simulink model "LAB_07_SIM_GG_SRP"  (R2022b)
settings: Solver=ode8  StartTime=0.0  StopTime=10000  FixedStep=0.05  RelTol=1e-3
values from neighbouring files (symbols this model uses):
  a = 16371e+3    (= 16371000)    [lab_07_MAT.m]
  A0 = diag([1 1 1])    [LAB_04_17_OCT_MAT_KIN.m]    (also in LAB_05_24_OCT_MAT_KIN_COSDIR.m; LAB_06.m = A_target_fun(0); core_attitude_test.m = eye(3,3); lab_07_MAT.m)
  A_B1 = 2e-2    (= 0.02)    [lab_07_MAT.m]
  A_B2 = 6e-2    (= 0.06)    [lab_07_MAT.m]
  A_B3 = 2e-2    (= 0.02)    [lab_07_MAT.m]
  A_B4 = 6e-2    (= 0.06)    [lab_07_MAT.m]
  A_B5 = 3e-2    (= 0.03)    [lab_07_MAT.m]
  A_B6 = 3e-2    (= 0.03)    [lab_07_MAT.m]
  A_P1 = 12e-2    (= 0.12)    [lab_07_MAT.m]
  A_P2 = 12e-2    (= 0.12)    [lab_07_MAT.m]
  A_P3 = 12e-2    (= 0.12)    [lab_07_MAT.m]
  A_P4 = 12e-2    (= 0.12)    [lab_07_MAT.m]
  ang = deg2rad(11.5)    [lab_07_MAT.m]
  e = 0    [lab_07_MAT.m]
  G = 6.67430e-11    (= 6.6743e-11)    [LAB_06.m]    (also in lab_07_MAT.m)
  g_1_0 = -29404.8    [lab_07_MAT.m]
  g_1_1 = -1450.9    [lab_07_MAT.m]
  h_1_1 = 4652.5    [lab_07_MAT.m]
  i = char('pippo')    [LAB_01_19_SEPT.m]    (also in lab_07_MAT.m = 0.1)
  I = [Ix 0 0 ... (first row only)    [LAB_03_3_OCT_MAT_EUL_2_VERIFICATION.m]    (also in LAB_03_3_OCT_MAT_EUL_DOUBLESPIN.m = diag([Ix, Iy, Iz]); LAB_03_3_OCT_MAT_EUL_SPINAXIS.m = diag([Ix, Iy, Iz]); LAB_03_3_OCT_MAT_EUL_VECT.m; LAB_04_17_OCT_MAT_KIN.m)
  j_B = [0.01; 0.05; 0.01]    [lab_07_MAT.m]
  Mt = 5.972e+24    [LAB_06.m]    (also in lab_07_MAT.m)
  N_B1 = [1,0,0]'    [lab_07_MAT.m]
  N_B2 = [0,1,0]'    [lab_07_MAT.m]
  N_B3 = [-1,0,0]'    [lab_07_MAT.m]
  N_B4 = [0,-1,0]'    [lab_07_MAT.m]
  N_B5 = [0,0,1]'    [lab_07_MAT.m]
  N_B6 = [0,0,-1]    [lab_07_MAT.m]
  N_P1 = [0,0,1]    [lab_07_MAT.m]
  N_P2 = [0,0,-1]    [lab_07_MAT.m]
  N_P3 = [0,0,1]    [lab_07_MAT.m]
  N_P4 = [0,0,-1]    [lab_07_MAT.m]
  n_rot = 0.0012    [lab_07_MAT.m]
  n_sun = 2*pi/T    (= 1.99238499086e-07)    [lab_07_MAT.m]
  om_0 = [om_x0, om_y0, om_z0]    [LAB_03_3_OCT_MAT_EUL.m]    (also in LAB_03_3_OCT_MAT_EUL_2_VERIFICATION.m = [om_x0; om_y0; om_z0]; LAB_03_3_OCT_MAT_EUL_DOUBLESPIN.m = [om_x0; om_y0; om_z0]; LAB_03_3_OCT_MAT_EUL_SPINAXIS.m = [om_x0; om_y0; om_z0]; LAB_03_3_OCT_MAT_EUL_VECT.m = [om_x0; om_y0; om_z0])
  om_target = [0; 0; n]    [LAB_06.m]    (also in lab_07_MAT.m)
  P = [Px, Py, Pz]    [LAB_03_3_OCT_MAT_EUL_VECT.m]    (also in lab_07_MAT.m = 4.52666666667e-06)
  R = 6.371e+6 + H    (= 6381000)    [LAB_06.m]    (also in lab_07_MAT.m = 6378000)
  r_B1 = 1e-2*[15,0,0]    [lab_07_MAT.m]
  r_B2 = 1e-2*[0,5,0]    [lab_07_MAT.m]
  r_B3 = 1e-2*[-15,0,0]    [lab_07_MAT.m]
  r_B4 = 1e-2*[0,-5,0]    [lab_07_MAT.m]
  r_B5 = 1e-2*[0,0,10]    [lab_07_MAT.m]
  r_B6 = 1e-2*[0,0,-10]    [lab_07_MAT.m]
  r_P1 = 1e-2*[0,20,10]    [lab_07_MAT.m]
  r_P2 = 1e-2*[0,20,10]    [lab_07_MAT.m]
  r_P3 = 1e-2*[0,-20,10]    [lab_07_MAT.m]
  r_P4 = 1e-2*[0,-20,10]    [lab_07_MAT.m]
  r_sun = 149597870000    [lab_07_MAT.m]
  rho_d = 0.1    [lab_07_MAT.m]
  rho_sB = 0.5    [lab_07_MAT.m]
  rho_sP = 0.5    [lab_07_MAT.m]
  rot_E = 7.29e-5    (= 7.29e-05)    [lab_07_MAT.m]
  theta_0 = 3/2 * pi    (= 4.71238898038)    [lab_07_MAT.m]
libraries: matrix_library x17, sharedutil x3, vrlib x1
(part 1 of 2)
settings Model: Creator=maria  LastModifiedBy=maria
settings OptimizationCC: BlockReduction=off  DefaultParameterBehavior=Inlined  BufferReuse=off

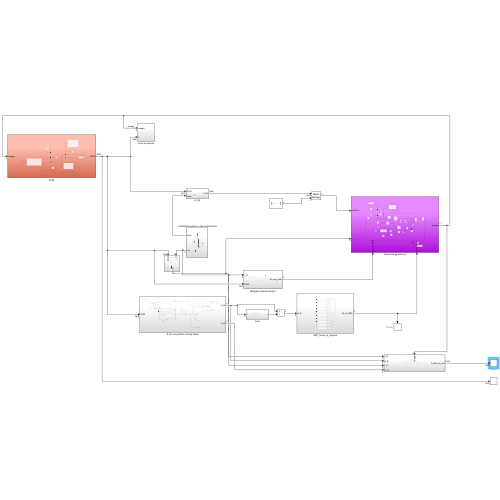
[thumbnail: Simulink's stored preview of the top-level diagram]
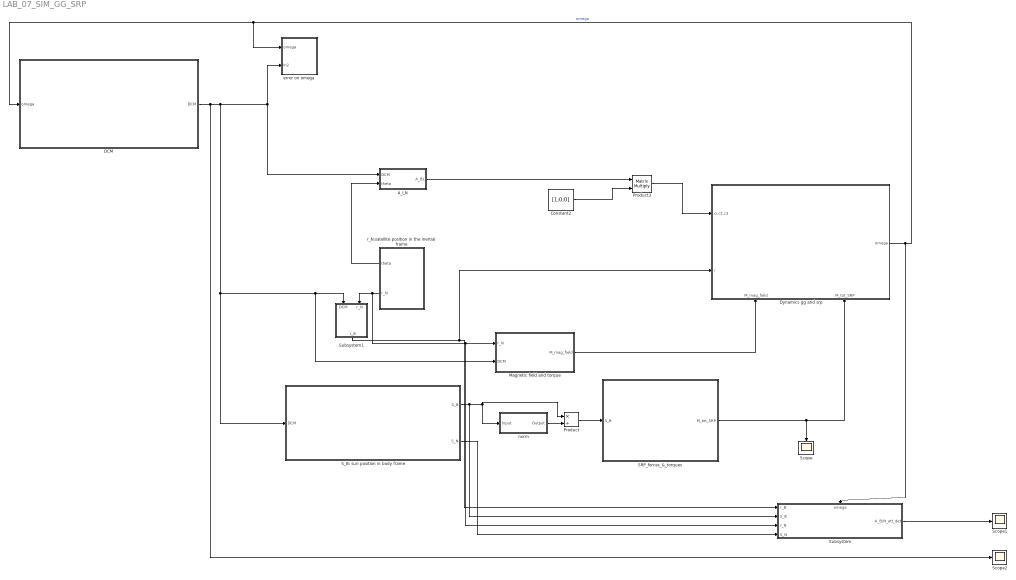
== system LAB_07_SIM_GG_SRP ==
  A_LN : Subsystem
  Constant2 : Constant  Value=[1;0;0]
  DCM : Subsystem
  Dynamics gg and srp : Subsystem
      settings: PortSchema="{\"entries\":[{\"content\":{\"sides\":[{\"content\":{\"connectorIds\":[\"In1\",\"In2\"]},\"type\":\"ConnectorPlacement.EquallySpacedRectSide\",\"uuid\":\"bc05948c-2cea-49c7-b73f-89081b27225b\"},{\"content\":{\"connectorIds\":[\"Out1\"],\"side\":\"RIGHT\"},\"type\":\"ConnectorPlacement.EquallySpacedRectSide\",\"uuid\":\"6a29747a-be53-4398-a7e6-b9c90b18bedd\"},{\"content\":{\"connectorIds\":[],\"side\":\"TOP\"},\"type\":\"ConnectorPlacement.EquallySpacedRectSide\",\"uuid\":\"b66eb14e-a712-4ddc-a917-1977d9025fb8\"},{\"content\":{\"connectorIds\":[\"In3\",\"In4\"],\"side\":\"BOTTOM\"},\"type\":\"ConnectorPlacement.EquallySpacedRectSide\",\"uuid\":\"2ac0e41d-d672-4d63-8cc6-d69981e4dca2\"}]},\"type\":\"ConnectorPlacement.EquallySpacedConnector\",\"uuid\":\"0ab2aa15-ff07-4137-9a78-1a42d8e85e1c\"}],\"packageUris\":[\"http://schema.mathworks.com/mf0/Connector/R2020b\"],\"version\":\"1.0\"}"
  Magnetic field and torque : Subsystem
  Product : Product  Inputs=*/
  Product3 : Product  Multiplication=Matrix(*)
  SRP_forces_&_torques : Subsystem
  S_B: sun position in body frame : Subsystem
  Scope : Scope
  Scope1 : Scope
  Scope2 : Scope
  Subsystem : Subsystem
      settings: PortSchema="{\"entries\":[{\"content\":{\"sides\":[{\"content\":{\"connectorIds\":[\"In1\",\"In2\",\"In3\",\"In4\"]},\"type\":\"ConnectorPlacement.EquallySpacedRectSide\",\"uuid\":\"1b4c40a5-3c0a-45e1-a855-6d56c967dca4\"},{\"content\":{\"connectorIds\":[\"Out1\"],\"side\":\"RIGHT\"},\"type\":\"ConnectorPlacement.EquallySpacedRectSide\",\"uuid\":\"ce0815a5-5ed5-4025-9107-00bd731c7882\"},{\"content\":{\"connectorIds\":[\"In5\"],\"side\":\"TOP\"},\"type\":\"ConnectorPlacement.EquallySpacedRectSide\",\"uuid\":\"c74c6876-9b03-4c6e-a93c-f68aec76813e\"}]},\"type\":\"ConnectorPlacement.EquallySpacedConnector\",\"uuid\":\"b7c608c1-7ac4-4db0-ac2d-ea1ef077d94d\"}],\"packageUris\":[\"http://schema.mathworks.com/mf0/Connector/R2020b\"],\"version\":\"1.0\"}"
  Subsystem1 : Subsystem
  error on omega : Subsystem
  norm : Subsystem
  r_N:satellite position in the inertial frame : Subsystem
  wires:
  Product/1 -> SRP_forces_&_torques/1(S_B)
  S_B: sun position in body frame/1(S_B) -> Subsystem/2(S_B), norm/1(Input), Product/1
  norm/1(Output) -> Product/2
  r_N:satellite position in the inertial frame/2(r_N) -> Subsystem/3(r_N), Magnetic field and torque/1(r_N), Subsystem1/2(r_N)
  DCM/1(DCM) -> Scope2/1, error on omega/2(In2), A_LN/1(DCM), S_B: sun position in body frame/1(DCM), Magnetic field and torque/2(DCM), Subsystem1/1(DCM)
  Product3/1 -> Dynamics gg and srp/1(ci,c2,c3)
  Subsystem1/1(r_B) -> Subsystem/1(r_B), Dynamics gg and srp/2(r)
  Constant2/1 -> Product3/2
  Dynamics gg and srp/1(omega) -> Subsystem/5(omega), error on omega/1(omega), DCM/1(omega)  "omega"
  A_LN/1(A_BL) -> Product3/1
  SRP_forces_&_torques/1(M_tot_SRP) -> Scope/1, Dynamics gg and srp/4(M_tot_SRP)
  r_N:satellite position in the inertial frame/1(theta) -> A_LN/2(theta)
  Magnetic field and torque/1(M_mag_field) -> Dynamics gg and srp/3(M_mag_field)
  S_B: sun position in body frame/2(S_N) -> Subsystem/4(S_N)
  Subsystem/1(A_B/N_att_det) -> Scope1/1

== system LAB_07_SIM_GG_SRP/A_LN ==
  DCM : Inport
  theta : Inport  Port=2
  Constant : Constant  Value=i
  Product1 : Product  Multiplication=Matrix(*)
  Product2 : Product  Multiplication=Matrix(*)
  Scope1 : Scope
  Subsystem : Subsystem
  Subsystem3 : Subsystem
  To Workspace : ToWorkspace  VariableName=A_LN  SampleTime=-1
  To Workspace2 : ToWorkspace  VariableName=error_A1  SampleTime=-1
  Transpose : Math  Operator=transpose
  A_BL : Outport
  wires:
  theta/1 -> Subsystem3/1(theta)
  Constant/1 -> Subsystem/1(i)
  Subsystem3/1(A_theta) -> Product1/1
  Subsystem/1(A_i) -> Product1/2
  Product2/1 -> To Workspace2/1, A_BL/1, Scope1/1
  Product1/1 -> Transpose/1, To Workspace/1
  DCM/1 -> Product2/1
  Transpose/1 -> Product2/2

== system LAB_07_SIM_GG_SRP/DCM ==
  note: A
  omega : Inport
  Determinant Chech fo Validation : Subsystem
  Gain1 : Gain  Gain=-1
  Integrator1 : Integrator  InitialCondition=A0
  Product2 : Product  Multiplication=Matrix(*)
  Scope1 : Scope
  Scope2 : Scope
  Subsystem : Subsystem
  To Workspace2 : ToWorkspace  VariableName=A  SampleTime=-1
  To Workspace3 : ToWorkspace  VariableName=A_dot  SampleTime=-1
  matrix of omega cross prod : Subsystem
  DCM : Outport
  wires:
  Integrator1/1 -> Subsystem/1(A1), Scope2/1, Determinant Chech fo Validation/1(DCM), DCM/1, To Workspace2/1
  matrix of omega cross prod/1(Out1) -> Product2/1
  Product2/1 -> Gain1/1  "A_dot"
  omega/1 -> matrix of omega cross prod/1(om)
  Gain1/1 -> Integrator1/1, To Workspace3/1, Scope1/1
  Subsystem/1(A_orthonormalized1) -> Product2/2

== system LAB_07_SIM_GG_SRP/Dynamics gg and srp ==
  ci,c2,c3 : Inport
  r : Inport  Port=2
  M_mag_field : Inport  Port=3
  M_tot_SRP : Inport  Port=4
  Constant : Constant  Value=I
  Constant1 : Constant  Value=I
  Constant2 : Constant  Value=G*Mt
  Constant3 : Constant  Value=3
  Cross Product : matrix_library/Cross Product
  Cross Product1 : matrix_library/Cross Product
  Gain : Gain  Gain=3
  Gain1 : Gain
  Gain2 : Gain
  Gain3 : Gain
  Integrator : Integrator  InitialCondition=om_0
  Power : Math  Operator=pow
  Product : Product  Multiplication=Matrix(*)
  Product1 : Product  Inputs=/*  Multiplication=Matrix(*)
  Product2 : Product  Multiplication=Matrix(*)
  Product3 : Product  Inputs=/*
  Product4 : Product
  Scope : Scope
  Scope1 : Scope
  Scope2 : Scope
  Sum : Sum  Inputs=+---
  To Workspace : ToWorkspace  VariableName=M_GG  SampleTime=-1
  To Workspace1 : ToWorkspace  VariableName=omega  SampleTime=-1
  To Workspace2 : ToWorkspace  VariableName=omega_dot  SampleTime=-1
  norm : Subsystem
  validation : Subsystem
  omega : Outport
  wires:
  Product1/1 -> Integrator/1, To Workspace2/1, Scope1/1  "om_dot"
  Product/1 -> Cross Product/1
  r/1 -> norm/1(Input)
  Constant1/1 -> Product2/1
  Cross Product/1 -> Sum/1
  Sum/1 -> Product1/2
  ci,c2,c3/1 -> Cross Product1/2, Product2/2
  Product2/1 -> Cross Product1/1
  Constant/1 -> validation/2(In2), Product1/1, Product/1  "I"
  Integrator/1 -> Product/2, Cross Product/2, validation/1(om), To Workspace1/1, Scope/1, omega/1  "om"
  Cross Product1/1 -> Product4/1
  Gain/1 -> Product4/2
  Product4/1 -> To Workspace/1, Gain2/1, Scope2/1  "M_gg"
  Product3/1 -> Gain/1
  M_tot_SRP/1 -> Gain1/1
  M_mag_field/1 -> Gain3/1
  Gain1/1 -> Sum/2
  Gain2/1 -> Sum/4
  norm/1(Output) -> Power/1
  Constant3/1 -> Power/2
  Power/1 -> Product3/1
  Constant2/1 -> Product3/2
  Gain3/1 -> Sum/3

== system LAB_07_SIM_GG_SRP/Magnetic field and torque ==
  r_N : Inport
  DCM : Inport  Port=2
  Constant : Constant  Value=j_B
  Constant10 : Constant  Value=3
  Constant5 : Constant  Value=R
  Constant9 : Constant  Value=3
  Cross Product : matrix_library/Cross Product
  Dot Product : DotProduct  OutDataTypeStr=Inherit: Inherit via internal rule
  Gain : Gain  Gain=1e-9
  Gain1 : Gain  Gain=3
  MatrixMultiply : Product  Multiplication=Matrix(*)
  Normalize Vector : vrlib/Utilities/Normalize Vector  maxzero=0
  Power : Math  Operator=pow
  Power1 : Math  Operator=pow
  Product3 : Product  Inputs=**/
  Product4 : Product
  Product5 : Product
  Scope : Scope
  Scope1 : Scope
  Scope3 : Scope
  Subsystem : Subsystem
  Sum1 : Sum  Inputs=-+
  To Workspace : ToWorkspace  VariableName=b_N  SampleTime=-1
  To Workspace1 : ToWorkspace  VariableName=M_Magfiel  SampleTime=-1
  To Workspace3 : ToWorkspace  VariableName=b_mag_field  SampleTime=-1
  m : Subsystem
  norm1 : Subsystem
  M_mag_field : Outport
  wires:
  r_N/1 -> Normalize Vector/1, norm1/1(Input)
  Constant5/1 -> Power/1
  Constant9/1 -> Power/2
  Power/1 -> Product3/2
  Constant10/1 -> Power1/2
  norm1/1(Output) -> Power1/1  "r_norm"
  Power1/1 -> Product3/3
  Product3/1 -> Product4/1
  Dot Product/1 -> Product5/1
  m/1(m) -> Sum1/1, Dot Product/1
  Normalize Vector/1 -> Product5/2, Dot Product/2
  Sum1/1 -> Product4/2
  Subsystem/1(H0) -> Gain/1
  Product4/1 -> MatrixMultiply/2, To Workspace/1, Scope/1
  MatrixMultiply/1 -> Cross Product/2, Scope3/1, To Workspace3/1  "b_B"
  DCM/1 -> MatrixMultiply/1
  Constant/1 -> Cross Product/1
  Cross Product/1 -> To Workspace1/1, Scope1/1, M_mag_field/1  "M_mag_field"
  Product5/1 -> Gain1/1
  Gain1/1 -> Sum1/2
  Gain/1 -> Product3/1

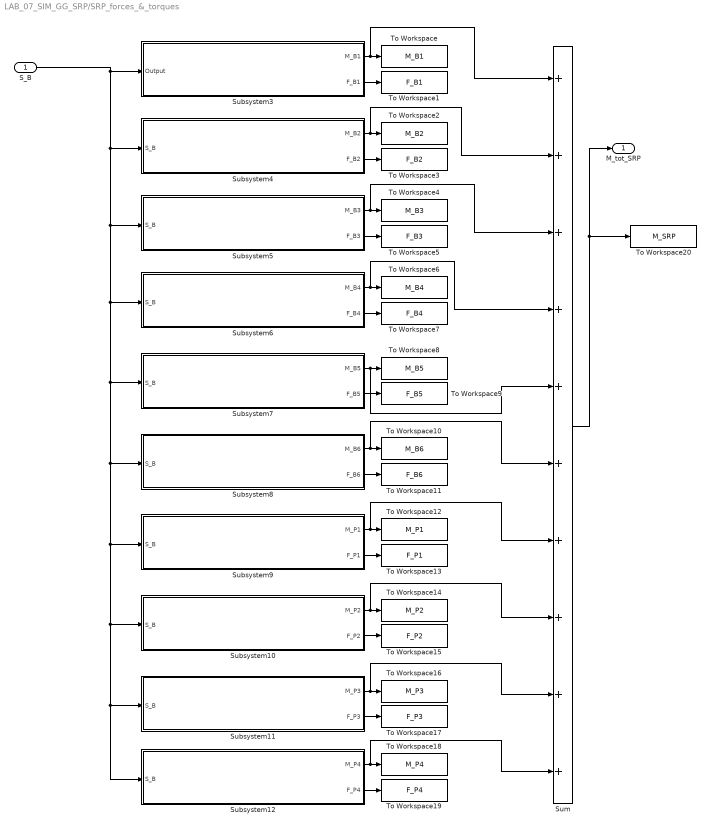
== system LAB_07_SIM_GG_SRP/SRP_forces_&_torques ==
  S_B : Inport
  Subsystem10 : Subsystem
  Subsystem11 : Subsystem
  Subsystem12 : Subsystem
  Subsystem3 : Subsystem
  Subsystem4 : Subsystem
  Subsystem5 : Subsystem
  Subsystem6 : Subsystem
  Subsystem7 : Subsystem
  Subsystem8 : Subsystem
  Subsystem9 : Subsystem
  Sum : Sum  Inputs=++++++++++
  To Workspace : ToWorkspace  VariableName=M_B1  SampleTime=-1
  To Workspace1 : ToWorkspace  VariableName=F_B1  SampleTime=-1
  To Workspace10 : ToWorkspace  VariableName=M_B6  SampleTime=-1
  To Workspace11 : ToWorkspace  VariableName=F_B6  SampleTime=-1
  To Workspace12 : ToWorkspace  VariableName=M_P1  SampleTime=-1
  To Workspace13 : ToWorkspace  VariableName=F_P1  SampleTime=-1
  To Workspace14 : ToWorkspace  VariableName=M_P2  SampleTime=-1
  To Workspace15 : ToWorkspace  VariableName=F_P2  SampleTime=-1
  To Workspace16 : ToWorkspace  VariableName=M_P3  SampleTime=-1
  To Workspace17 : ToWorkspace  VariableName=F_P3  SampleTime=-1
  To Workspace18 : ToWorkspace  VariableName=M_P4  SampleTime=-1
  To Workspace19 : ToWorkspace  VariableName=F_P4  SampleTime=-1
  To Workspace2 : ToWorkspace  VariableName=M_B2  SampleTime=-1
  To Workspace20 : ToWorkspace  VariableName=M_SRP  SampleTime=-1
  To Workspace3 : ToWorkspace  VariableName=F_B2  SampleTime=-1
  To Workspace4 : ToWorkspace  VariableName=M_B3  SampleTime=-1
  To Workspace5 : ToWorkspace  VariableName=F_B3  SampleTime=-1
  To Workspace6 : ToWorkspace  VariableName=M_B4  SampleTime=-1
  To Workspace7 : ToWorkspace  VariableName=F_B4  SampleTime=-1
  To Workspace8 : ToWorkspace  VariableName=M_B5  SampleTime=-1
  To Workspace9 : ToWorkspace  VariableName=F_B5  SampleTime=-1
  M_tot_SRP : Outport
  wires:
  S_B/1 -> Subsystem11/1(S_B), Subsystem12/1(S_B), Subsystem10/1(S_B), Subsystem9/1(S_B), Subsystem8/1(S_B), Subsystem7/1(S_B), Subsystem6/1(S_B), Subsystem5/1(S_B), Subsystem4/1(S_B), Subsystem3/1(Output)
  Subsystem7/2(F_B5) -> To Workspace9/1
  Subsystem12/2(F_P4) -> To Workspace19/1
  Subsystem12/1(M_P4) -> Sum/10, To Workspace18/1
  Subsystem6/1(M_B4) -> Sum/4, To Workspace6/1
  Subsystem7/1(M_B5) -> Sum/5, To Workspace8/1
  Subsystem8/1(M_B6) -> Sum/6, To Workspace10/1
  Subsystem10/2(F_P2) -> To Workspace15/1
  Subsystem11/1(M_P3) -> Sum/9, To Workspace16/1
  Subsystem10/1(M_P2) -> Sum/8, To Workspace14/1
  Subsystem3/2(F_B1) -> To Workspace1/1
  Subsystem9/2(F_P1) -> To Workspace13/1
  Subsystem4/1(M_B2) -> Sum/2, To Workspace2/1
  Subsystem5/1(M_B3) -> Sum/3, To Workspace4/1
  Subsystem11/2(F_P3) -> To Workspace17/1
  Subsystem5/2(F_B3) -> To Workspace5/1
  Subsystem3/1(M_B1) -> Sum/1, To Workspace/1
  Subsystem8/2(F_B6) -> To Workspace11/1
  Subsystem6/2(F_B4) -> To Workspace7/1
  Subsystem4/2(F_B2) -> To Workspace3/1
  Subsystem9/1(M_P1) -> Sum/7, To Workspace12/1
  Sum/1 -> M_tot_SRP/1, To Workspace20/1

== system LAB_07_SIM_GG_SRP/S_B: sun position in body frame ==
  DCM : Inport
  Clock : Clock
  Constant6 : Constant  Value=n_sun
  Constant7 : Constant  Value=eps
  Constant8 : Constant  Value=eps
  Constant9 : Constant  Value=r_sun
  Cos4 : Trigonometry  Operator=cos
  Cos5 : Trigonometry  Operator=cos
  MatrixMultiply1 : Product  Multiplication=Matrix(*)
  Mux1 : Mux  Inputs=3
  Product{5..8} (4 alike) : Product
  Scope4 : Scope
  Scope6 : Scope
  Sin2 : Trigonometry
  Sin3 : Trigonometry
  Sin4 : Trigonometry
  To Workspace4 : ToWorkspace  VariableName=time  SampleTime=-1
  To Workspace5 : ToWorkspace  VariableName=simout1  SaveFormat=Timeseries  SampleTime=-1
  To Workspace6 : ToWorkspace  VariableName=S_B  SampleTime=-1
  S_B : Outport
  S_N : Outport  Port=2
  wires:
  Sin2/1 -> Product6/1
  Product8/1 -> S_N/1, MatrixMultiply1/2, To Workspace5/1, Scope4/1
  MatrixMultiply1/1 -> S_B/1, To Workspace6/1, Scope6/1  "S_B"
  Constant7/1 -> Cos5/1
  Constant8/1 -> Sin4/1
  Sin3/1 -> Product7/1
  DCM/1 -> MatrixMultiply1/1
  Product7/1 -> Mux1/3
  Constant6/1 -> Product5/2
  Cos5/1 -> Product6/2
  Mux1/1 -> Product8/2
  Constant9/1 -> Product8/1
  Clock/1 -> Product5/1, To Workspace4/1
  Product5/1 -> Sin3/1, Sin2/1, Cos4/1
  Product6/1 -> Mux1/2
  Cos4/1 -> Mux1/1
  Sin4/1 -> Product7/2

== system LAB_07_SIM_GG_SRP/Subsystem ==
  r_B : Inport
  S_B : Inport  Port=2
  r_N : Inport  Port=3
  S_N : Inport  Port=4
  omega : Inport  Port=5
  Check_Orthogonality_S : Subsystem
  Check_Orthogonality_V : Subsystem
  Constant : Constant
  Constant1 : Constant
  Cross Product{,1..3} (4 alike) : matrix_library/Cross Product
  DCM : Subsystem
  Determinant of 3x3 Matrix : sharedutil/Determinant of 3x3 Matrix  aMode=aMode
      settings: LibrarySourceBlock=|
      | aerolibutil/Determinant of
      | 3x3 Matrix
  Matrix Concatenate : Concatenate  NumInputs=3  Mode=Multidimensional array  ConcatenateDimension=2
  Matrix Concatenate1 : Concatenate  NumInputs=3  Mode=Multidimensional array  ConcatenateDimension=2
  MatrixMultiply : Product  Multiplication=Matrix(*)
  OR : Logic  Operator=OR  IconShape=distinctive  AllPortsSameDT=off  OutDataTypeStr=boolean
  Product : Product  Inputs=*/
  Product1 : Product  Inputs=*/
  Scope : Scope
  Scope1 : Scope
  Scope2 : Scope
  Switch : Switch  Criteria=u2 ~= 0  SaturateOnIntegerOverflow=off  InputSameDT=off
  Switch1 : Switch  Criteria=u2 ~= 0  SaturateOnIntegerOverflow=off  InputSameDT=off
  Switch2 : Switch  Criteria=u2 ~= 0  SaturateOnIntegerOverflow=off  InputSameDT=off
  Transpose : Math  Operator=transpose
  norm : Subsystem
  norm1 : Subsystem
  A_B/N_att_det : Outport
  wires:
  r_B/1 -> Matrix Concatenate/1, Cross Product1/1, Cross Product/1  "s1"
  S_B/1 -> Cross Product/2
  Cross Product/1 -> Product/1, norm/1(Input)
  norm/1(Output) -> OR/1, Switch/2, Switch/1
  Product/1 -> Matrix Concatenate/2, Cross Product1/2  "s2"
  Cross Product1/1 -> Matrix Concatenate/3  "s3"
  Matrix Concatenate/1 -> Scope/1, Check_Orthogonality_S/1(S), MatrixMultiply/1  "S"
  Cross Product3/1 -> Matrix Concatenate1/3  "s3"
  Matrix Concatenate1/1 -> Check_Orthogonality_V/1(V), Scope1/1, Transpose/1  "V"
  r_N/1 -> Cross Product2/1, Matrix Concatenate1/1, Cross Product3/1  "s1"
  S_N/1 -> Cross Product2/2
  Cross Product2/1 -> Product1/1, norm1/1(Input)
  Product1/1 -> Matrix Concatenate1/2, Cross Product3/2  "s2"
  Transpose/1 -> MatrixMultiply/2
  MatrixMultiply/1 -> Switch2/1, Determinant of 3x3 Matrix/1
  Determinant of 3x3 Matrix/1 -> Scope2/1
  Constant/1 -> Switch/3
  Switch/1 -> Product/2
  Switch1/1 -> Product1/2
  Constant1/1 -> Switch1/3
  norm1/1(Output) -> OR/2, Switch1/2, Switch1/1
  omega/1 -> DCM/1(omega)
  Switch2/1 -> A_B/N_att_det/1
  OR/1 -> Switch2/2

== system LAB_07_SIM_GG_SRP/Subsystem1 ==
  DCM : Inport
  r_N : Inport  Port=2
  MatrixMultiply : Product  Multiplication=Matrix(*)
  Scope3 : Scope
  To Workspace3 : ToWorkspace  VariableName=r_B  SampleTime=-1
  r_B : Outport
  wires:
  MatrixMultiply/1 -> r_B/1, To Workspace3/1, Scope3/1  "r_B"
  r_N/1 -> MatrixMultiply/2
  DCM/1 -> MatrixMultiply/1

== system LAB_07_SIM_GG_SRP/error on omega ==
  omega : Inport
  In2 : Inport  Port=2
  Constant : Constant  Value=om_target
  Product1 : Product  Multiplication=Matrix(*)
  Scope : Scope
  Sum : Sum  Inputs=+-
  To Workspace : ToWorkspace  VariableName=error_omega  SampleTime=-1
  wires:
  Sum/1 -> To Workspace/1, Scope/1
  Product1/1 -> Sum/2
  In2/1 -> Product1/1
  Constant/1 -> Product1/2
  omega/1 -> Sum/1

== system LAB_07_SIM_GG_SRP/norm ==
  Input : Inport
  Demux : Demux  Outputs=3
  Sqrt : Sqrt
  Square : Math  Operator=square
  Square1 : Math  Operator=square
  Square2 : Math  Operator=square
  Sum : Sum  Inputs=+++
  Output : Outport
  wires:
  Square/1 -> Sum/1
  Square1/1 -> Sum/2
  Square2/1 -> Sum/3
  Sum/1 -> Sqrt/1
  Input/1 -> Demux/1
  Sqrt/1 -> Output/1
  Demux/1 -> Square/1
  Demux/2 -> Square1/1
  Demux/3 -> Square2/1

== system LAB_07_SIM_GG_SRP/r_N:satellite position in the inertial frame ==
  Constant : Constant
  Constant1 : Constant  Value=n_rot
  Constant2 : Constant  Value=(1-e^2)^(3/2)
  Constant3 : Constant  Value=a
  Constant4 : Constant  Value=(1-e^2)
  Constant5 : Constant  Value=i
  Cos : Trigonometry  Operator=cos
  Cos1 : Trigonometry  Operator=cos
  Cos2 : Trigonometry  Operator=cos
  Cos3 : Trigonometry
  Gain1 : Gain  Gain=e
  Integrator : Integrator  InitialCondition=theta_0  WrapState=on  WrappedStateUpperValue=2*pi  WrappedStateLowerValue=0
  Mux : Mux  Inputs=3
  Product : Product  Inputs=**/
  Product1 : Product  Inputs=**/
  Product2 : Product
  Product3 : Product
  Product4 : Product
  Scope : Scope
  Scope1 : Scope
  Scope2 : Scope
  Sin : Trigonometry
  Sin1 : Trigonometry
  Square : Math  Operator=square
  Sum : Sum
  To Workspace : ToWorkspace  VariableName=r_N  SampleTime=-1
  To Workspace1 : ToWorkspace  VariableName=theta  SampleTime=-1
  To Workspace2 : ToWorkspace  VariableName=simout  SaveFormat=Timeseries  SampleTime=-1
  theta : Outport
  r_N : Outport  Port=2
  wires:
  Product2/1 -> Mux/2
  Sin1/1 -> Product2/1
  Constant/1 -> Sum/1
  Integrator/1 -> Scope1/1, To Workspace1/1, Cos2/1, Sin1/1, Cos3/1, theta/1, Cos/1  "theta"
  Product3/1 -> r_N/1, To Workspace/1, Scope/1
  Constant1/1 -> Product/1
  Sin/1 -> Product4/2
  Constant5/1 -> Cos1/1, Sin/1
  Cos3/1 -> Product4/1
  Constant3/1 -> Product1/1
  Square/1 -> Product/2
  Gain1/1 -> Sum/2
  Cos1/1 -> Product2/2
  Sum/1 -> Product1/3, Square/1
  Product/1 -> Integrator/1  "theta_dot"
  Cos/1 -> Gain1/1
  Product4/1 -> Mux/3
  Cos2/1 -> Mux/1
  Mux/1 -> Product3/2  "r_N"
  Constant2/1 -> Product/3
  Product1/1 -> To Workspace2/1, Scope2/1, Product3/1  "r"
  Constant4/1 -> Product1/2

== system LAB_07_SIM_GG_SRP/A_LN/Subsystem ==
  i : Inport
  Constant{,3,6..7} (4 alike) : Constant  Value=0
  Constant4 : Constant
  Cos2 : Trigonometry  Operator=cos
  Cos4 : Trigonometry  Operator=cos
  Gain1 : Gain  Gain=-1
  Matrix Concatenate1 : Concatenate  NumInputs=3  Mode=Multidimensional array
  Mux2 : Mux  Inputs=3
  Mux3 : Mux  Inputs=3
  Mux4 : Mux  Inputs=3
  Sin3 : Trigonometry
  Sin4 : Trigonometry
  Transpose2 : Math  Operator=transpose
  Transpose3 : Math  Operator=transpose
  Transpose4 : Math  Operator=transpose
  A_i : Outport
  wires:
  Constant/1 -> Mux2/3
  Mux2/1 -> Transpose2/1
  Constant3/1 -> Mux2/2
  Constant4/1 -> Mux2/1
  Transpose2/1 -> Matrix Concatenate1/1
  Cos2/1 -> Mux3/2
  Mux3/1 -> Transpose3/1
  Sin3/1 -> Mux3/3
  Constant6/1 -> Mux3/1
  Transpose3/1 -> Matrix Concatenate1/2
  Sin4/1 -> Mux4/2
  Cos4/1 -> Mux4/3
  Transpose4/1 -> Matrix Concatenate1/3
  Constant7/1 -> Mux4/1
  Mux4/1 -> Transpose4/1
  i/1 -> Cos4/1, Gain1/1, Sin3/1, Cos2/1
  Gain1/1 -> Sin4/1
  Matrix Concatenate1/1 -> A_i/1

== system LAB_07_SIM_GG_SRP/A_LN/Subsystem3 ==
  theta : Inport
  Constant : Constant
  Constant{1..4} (4 alike) : Constant  Value=0
  Cos : Trigonometry  Operator=cos
  Cos1 : Trigonometry  Operator=cos
  Gain : Gain  Gain=-1
  Matrix Concatenate : Concatenate  NumInputs=3  Mode=Multidimensional array
  Mux : Mux  Inputs=3
  Mux1 : Mux  Inputs=3
  Mux2 : Mux  Inputs=3
  Sin : Trigonometry
  Sin1 : Trigonometry
  Transpose : Math  Operator=transpose
  Transpose1 : Math  Operator=transpose
  Transpose2 : Math  Operator=transpose
  A_theta : Outport
  wires:
  theta/1 -> Cos1/1, Gain/1, Sin/1, Cos/1
  Cos/1 -> Mux/1
  Sin/1 -> Mux/2
  Constant1/1 -> Mux/3
  Matrix Concatenate/1 -> A_theta/1
  Mux/1 -> Transpose/1
  Gain/1 -> Sin1/1
  Sin1/1 -> Mux1/1
  Cos1/1 -> Mux1/2
  Constant2/1 -> Mux1/3
  Mux1/1 -> Transpose1/1
  Constant3/1 -> Mux2/2
  Constant/1 -> Mux2/3
  Constant4/1 -> Mux2/1
  Mux2/1 -> Transpose2/1
  Transpose/1 -> Matrix Concatenate/1
  Transpose1/1 -> Matrix Concatenate/2
  Transpose2/1 -> Matrix Concatenate/3

== system LAB_07_SIM_GG_SRP/DCM/Determinant Chech fo Validation ==
  DCM : Inport
  Determinant of 3x3 Matrix : sharedutil/Determinant of 3x3 Matrix  aMode=aMode
      settings: LibrarySourceBlock=|
      | aerolibutil/Determinant of
      | 3x3 Matrix
  MATLAB Function : MATLAB Function  TreatAsAtomicUnit=on
  To Workspace : ToWorkspace  VariableName=perpendicularity_flag  SampleTime=-1
  To Workspace4 : ToWorkspace  VariableName=detA  SampleTime=-1
  determinant : Scope
  perpendicularity : Scope
  wires:
  Determinant of 3x3 Matrix/1 -> determinant/1, To Workspace4/1
  DCM/1 -> MATLAB Function/1(DCM), Determinant of 3x3 Matrix/1
  MATLAB Function/1(perpendicularity_flag) -> To Workspace/1, perpendicularity/1

== system LAB_07_SIM_GG_SRP/DCM/Subsystem ==
  A1 : Inport
  Gain : Gain  Gain=1.5
  Gain1 : Gain  Gain=-0.5
  Gain4 : Gain  Commented=on  Gain=3/2
  Gain5 : Gain  Commented=on  Gain=1/2
  Product : Product  Inputs=3  Multiplication=Matrix(*)
  Product3 : Product  Commented=on  Inputs=3  Multiplication=Matrix(*)
  Sum : Sum  Commented=on  Inputs=+-
  Sum1 : Sum
  Transpose : Math  Commented=on  Operator=transpose
  Transpose1 : Math  Operator=transpose
  A_orthonormalized1 : Outport
  wires:
  Sum/1 -> ?
  Gain5/1 -> Sum/2
  Product3/1 -> Gain5/1
  Transpose/1 -> Product3/2  "A_transpose"
  Gain4/1 -> Sum/1
  A1/1 -> Product/1, Transpose1/1, Product/3, Gain/1
  Gain/1 -> Sum1/2
  Sum1/1 -> A_orthonormalized1/1
  Gain1/1 -> Sum1/1
  Product/1 -> Gain1/1
  Transpose1/1 -> Product/2

== system LAB_07_SIM_GG_SRP/DCM/matrix of omega cross prod ==
  om : Inport
  Constant1 : Constant  Value=0
  Constant2 : Constant  Value=0
  Constant3 : Constant  Value=0
  Demux : Demux  Outputs=3
  Display : Display
  Gain : Gain  Gain=-1
  Gain1 : Gain  Gain=-1
  Gain2 : Gain  Gain=-1
  Matrix Concatenate : Concatenate  NumInputs=3  Mode=Multidimensional array
  Mux : Mux  Inputs=3
  Mux1 : Mux  Inputs=3
  Mux2 : Mux  Inputs=3
  Scope : Scope
  Transpose : Math  Operator=transpose
  Transpose1 : Math  Operator=transpose
  Transpose2 : Math  Operator=transpose
  Out1 : Outport
  wires:
  Matrix Concatenate/1 -> Display/1, Scope/1, Out1/1
  Demux/1 -> Gain1/1, Mux2/2
  Mux1/1 -> Transpose1/1
  Constant3/1 -> Mux2/3
  Gain/1 -> Mux/2
  Gain2/1 -> Mux2/1
  Constant1/1 -> Mux/1
  Demux/3 -> Gain/1, Mux1/1
  Demux/2 -> Mux/3, Gain2/1
  Mux/1 -> Transpose/1
  Gain1/1 -> Mux1/3
  Mux2/1 -> Transpose2/1
  Constant2/1 -> Mux1/2
  om/1 -> Demux/1
  Transpose/1 -> Matrix Concatenate/1
  Transpose1/1 -> Matrix Concatenate/2
  Transpose2/1 -> Matrix Concatenate/3

== system LAB_07_SIM_GG_SRP/Dynamics gg and srp/norm ==
  Input : Inport
  Demux : Demux  Outputs=3
  Sqrt : Sqrt
  Square : Math  Operator=square
  Square1 : Math  Operator=square
  Square2 : Math  Operator=square
  Sum : Sum  Inputs=+++
  Output : Outport
  wires:
  Square/1 -> Sum/1
  Square1/1 -> Sum/2
  Square2/1 -> Sum/3
  Sum/1 -> Sqrt/1
  Input/1 -> Demux/1
  Sqrt/1 -> Output/1
  Demux/1 -> Square/1
  Demux/2 -> Square1/1
  Demux/3 -> Square2/1

== system LAB_07_SIM_GG_SRP/Dynamics gg and srp/validation ==
  om : Inport
  In2 : Inport  Port=2
  Gain : Gain  Gain=1/2
  Product : Product  Inputs=3  Multiplication=Matrix(*)
  Product2 : Product  Multiplication=Matrix(*)
  Scope : Scope
  Scope1 : Scope
  To Workspace : ToWorkspace  VariableName=E  SampleTime=-1
  To Workspace2 : ToWorkspace  VariableName=hnorm  SampleTime=-1
  Transpose1 : Math  Operator=transpose
  norm : Subsystem
  wires:
  Product2/1 -> norm/1(Input)
  norm/1(Output) -> To Workspace2/1, Scope1/1
  om/1 -> Transpose1/1, Product/3, Product2/2
  In2/1 -> Product/2, Product2/1  "I"
  Transpose1/1 -> Product/1
  Product/1 -> Gain/1
  Gain/1 -> Scope/1, To Workspace/1

== system LAB_07_SIM_GG_SRP/Magnetic field and torque/Subsystem ==
  Constant6 : Constant  Value=g_1_0
  Constant7 : Constant  Value=g_1_1
  Constant8 : Constant  Value=h_1_1
  Sqrt : Sqrt
  Square : Math  Operator=square
  Square1 : Math  Operator=square
  Square2 : Math  Operator=square
  Sum : Sum  Inputs=+++
  H0 : Outport
  wires:
  Constant8/1 -> Square2/1
  Square2/1 -> Sum/3
  Constant6/1 -> Square/1
  Constant7/1 -> Square1/1
  Square/1 -> Sum/1
  Sum/1 -> Sqrt/1
  Sqrt/1 -> H0/1  "H0"
  Square1/1 -> Sum/2

== system LAB_07_SIM_GG_SRP/Magnetic field and torque/m ==
  Clock : Clock
  Constant : Constant  Value=ang
  Constant2 : Constant  Value=rot_E
  Constant3 : Constant  Value=ang
  Constant4 : Constant  Value=ang
  Cos : Trigonometry  Operator=cos
  Cos1 : Trigonometry  Operator=cos
  Mux : Mux  Inputs=3
  Product : Product
  Product1 : Product
  Product2 : Product
  Scope : Scope
  Sin : Trigonometry
  Sin1 : Trigonometry
  Sin2 : Trigonometry
  norm : Subsystem
  m : Outport
  wires:
  Cos1/1 -> Product1/1
  Constant3/1 -> Sin1/1
  Product/1 -> Sin2/1, Cos1/1
  Constant/1 -> Sin/1
  Constant4/1 -> Cos/1
  Mux/1 -> m/1, norm/1(Input)  "m"
  Sin2/1 -> Product2/1
  Product2/1 -> Mux/2
  Constant2/1 -> Product/1
  Product1/1 -> Mux/1
  Sin1/1 -> Product2/2
  Clock/1 -> Product/2
  Sin/1 -> Product1/2
  Cos/1 -> Mux/3
  norm/1(Output) -> Scope/1

== system LAB_07_SIM_GG_SRP/Magnetic field and torque/norm1 ==
  Input : Inport
  Demux : Demux  Outputs=3
  Sqrt : Sqrt
  Square : Math  Operator=square
  Square1 : Math  Operator=square
  Square2 : Math  Operator=square
  Sum : Sum  Inputs=+++
  Output : Outport
  wires:
  Square/1 -> Sum/1
  Square1/1 -> Sum/2
  Square2/1 -> Sum/3
  Sum/1 -> Sqrt/1
  Input/1 -> Demux/1
  Sqrt/1 -> Output/1
  Demux/1 -> Square/1
  Demux/2 -> Square1/1
  Demux/3 -> Square2/1

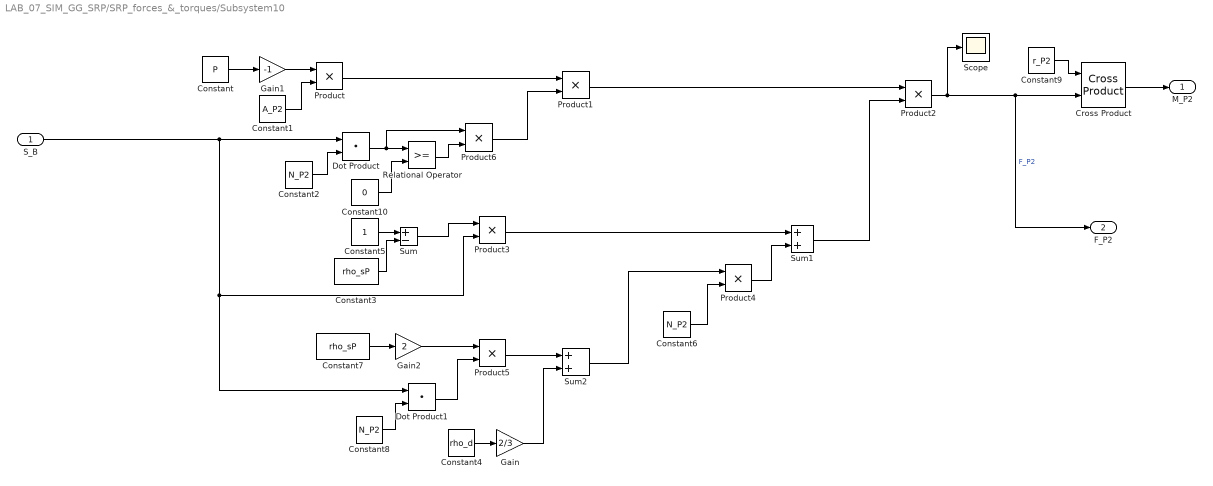
== system LAB_07_SIM_GG_SRP/SRP_forces_&_torques/Subsystem10 ==
  S_B : Inport
  Constant : Constant  Value=P
  Constant1 : Constant  Value=A_P2
  Constant10 : Constant  Value=0
  Constant2 : Constant  Value=N_P2
  Constant3 : Constant  Value=rho_sP
  Constant4 : Constant  Value=rho_d
  Constant5 : Constant
  Constant6 : Constant  Value=N_P2
  Constant7 : Constant  Value=rho_sP
  Constant8 : Constant  Value=N_P2
  Constant9 : Constant  Value=r_P2
  Cross Product : matrix_library/Cross Product
  Dot Product : DotProduct  OutDataTypeStr=Inherit: Inherit via internal rule
  Dot Product1 : DotProduct  OutDataTypeStr=Inherit: Inherit via internal rule
  Gain : Gain  Gain=2/3
  Gain1 : Gain  Gain=-1
  Gain2 : Gain  Gain=2
  Product{,1..6} (7 alike) : Product
  Relational Operator : RelationalOperator  OutDataTypeStr=boolean  RndMeth=Simplest  InputSameDT=off
  Scope : Scope
  Sum : Sum  Inputs=+-
  Sum1 : Sum
  Sum2 : Sum
  M_P2 : Outport
  F_P2 : Outport  Port=2
  wires:
  Sum1/1 -> Product2/2
  Constant4/1 -> Gain/1
  Product/1 -> Product1/1
  Constant3/1 -> Sum/2
  Constant5/1 -> Sum/1
  Constant9/1 -> Cross Product/1
  Gain1/1 -> Product/1
  Dot Product1/1 -> Product5/2
  Product3/1 -> Sum1/1
  Cross Product/1 -> M_P2/1
  Constant1/1 -> Product/2
  Sum2/1 -> Product4/1
  Constant7/1 -> Gain2/1
  Constant/1 -> Gain1/1
  Gain2/1 -> Product5/1
  Gain/1 -> Sum2/2
  Constant2/1 -> Dot Product/2
  Product1/1 -> Product2/1
  Sum/1 -> Product3/1
  Constant6/1 -> Product4/2
  Constant8/1 -> Dot Product1/2
  Product4/1 -> Sum1/2
  Product5/1 -> Sum2/1
  Product2/1 -> Scope/1, Cross Product/2, F_P2/1  "F_P2"
  S_B/1 -> Product3/2, Dot Product1/1, Dot Product/1
  Constant10/1 -> Relational Operator/2
  Relational Operator/1 -> Product6/2
  Dot Product/1 -> Product6/1, Relational Operator/1
  Product6/1 -> Product1/2

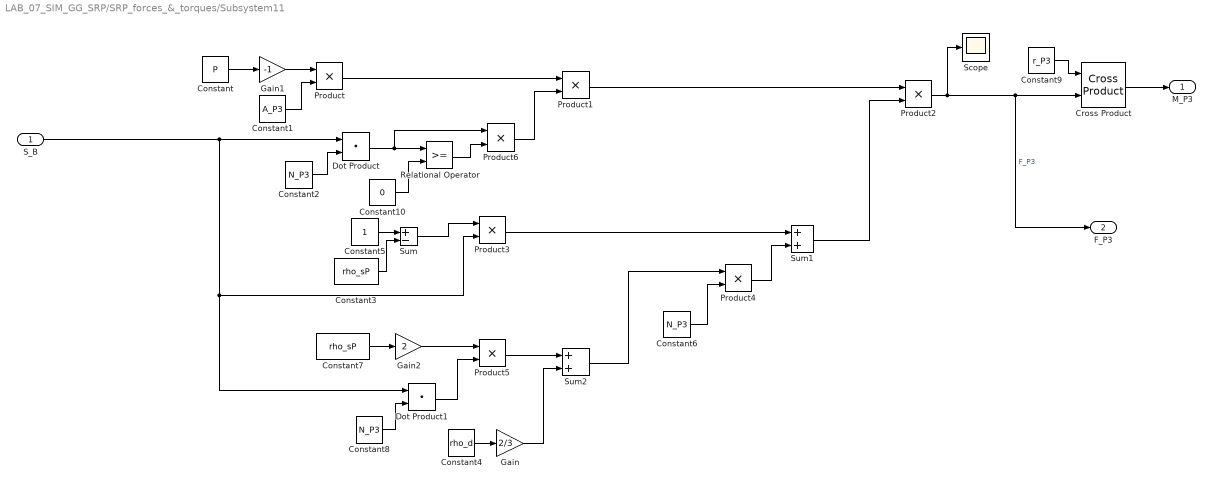
== system LAB_07_SIM_GG_SRP/SRP_forces_&_torques/Subsystem11 ==
  S_B : Inport
  Constant : Constant  Value=P
  Constant1 : Constant  Value=A_P3
  Constant10 : Constant  Value=0
  Constant2 : Constant  Value=N_P3
  Constant3 : Constant  Value=rho_sP
  Constant4 : Constant  Value=rho_d
  Constant5 : Constant
  Constant6 : Constant  Value=N_P3
  Constant7 : Constant  Value=rho_sP
  Constant8 : Constant  Value=N_P3
  Constant9 : Constant  Value=r_P3
  Cross Product : matrix_library/Cross Product
  Dot Product : DotProduct  OutDataTypeStr=Inherit: Inherit via internal rule
  Dot Product1 : DotProduct  OutDataTypeStr=Inherit: Inherit via internal rule
  Gain : Gain  Gain=2/3
  Gain1 : Gain  Gain=-1
  Gain2 : Gain  Gain=2
  Product{,1..6} (7 alike) : Product
  Relational Operator : RelationalOperator  OutDataTypeStr=boolean  RndMeth=Simplest  InputSameDT=off
  Scope : Scope
  Sum : Sum  Inputs=+-
  Sum1 : Sum
  Sum2 : Sum
  M_P3 : Outport
  F_P3 : Outport  Port=2
  wires:
  S_B/1 -> Dot Product/1, Dot Product1/1, Product3/2
  Product2/1 -> F_P3/1, Cross Product/2, Scope/1  "F_P3"
  Product5/1 -> Sum2/1
  Product4/1 -> Sum1/2
  Constant8/1 -> Dot Product1/2
  Constant6/1 -> Product4/2
  Sum/1 -> Product3/1
  Product1/1 -> Product2/1
  Constant2/1 -> Dot Product/2
  Gain/1 -> Sum2/2
  Gain2/1 -> Product5/1
  Constant/1 -> Gain1/1
  Constant7/1 -> Gain2/1
  Sum2/1 -> Product4/1
  Constant1/1 -> Product/2
  Cross Product/1 -> M_P3/1
  Product3/1 -> Sum1/1
  Dot Product1/1 -> Product5/2
  Gain1/1 -> Product/1
  Constant9/1 -> Cross Product/1
  Constant5/1 -> Sum/1
  Constant3/1 -> Sum/2
  Product/1 -> Product1/1
  Constant4/1 -> Gain/1
  Sum1/1 -> Product2/2
  Constant10/1 -> Relational Operator/2
  Relational Operator/1 -> Product6/2
  Dot Product/1 -> Product6/1, Relational Operator/1
  Product6/1 -> Product1/2

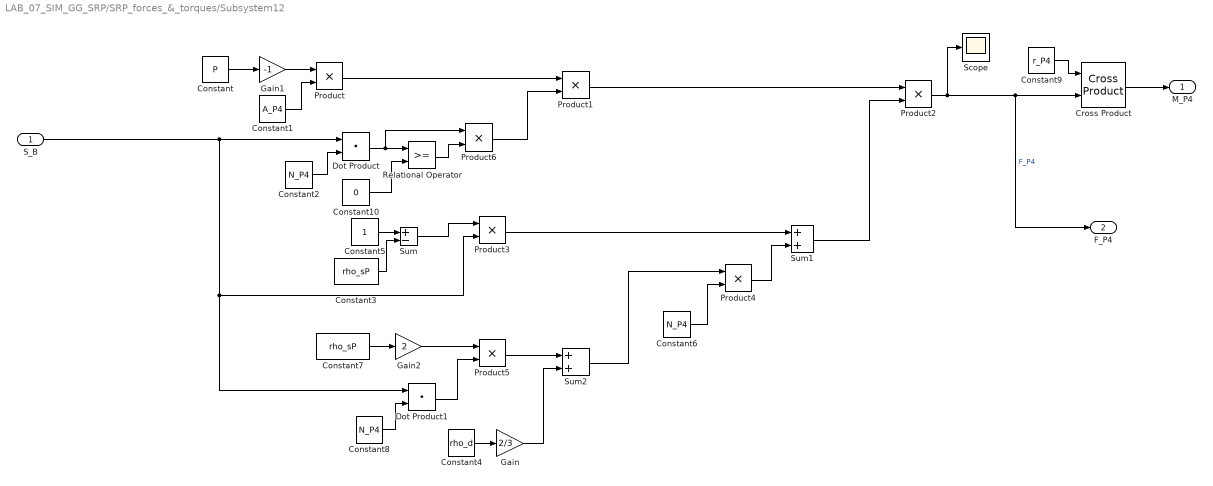
== system LAB_07_SIM_GG_SRP/SRP_forces_&_torques/Subsystem12 ==
  S_B : Inport
  Constant : Constant  Value=P
  Constant1 : Constant  Value=A_P4
  Constant10 : Constant  Value=0
  Constant2 : Constant  Value=N_P4
  Constant3 : Constant  Value=rho_sP
  Constant4 : Constant  Value=rho_d
  Constant5 : Constant
  Constant6 : Constant  Value=N_P4
  Constant7 : Constant  Value=rho_sP
  Constant8 : Constant  Value=N_P4
  Constant9 : Constant  Value=r_P4
  Cross Product : matrix_library/Cross Product
  Dot Product : DotProduct  OutDataTypeStr=Inherit: Inherit via internal rule
  Dot Product1 : DotProduct  OutDataTypeStr=Inherit: Inherit via internal rule
  Gain : Gain  Gain=2/3
  Gain1 : Gain  Gain=-1
  Gain2 : Gain  Gain=2
  Product{,1..6} (7 alike) : Product
  Relational Operator : RelationalOperator  OutDataTypeStr=boolean  RndMeth=Simplest  InputSameDT=off
  Scope : Scope
  Sum : Sum  Inputs=+-
  Sum1 : Sum
  Sum2 : Sum
  M_P4 : Outport
  F_P4 : Outport  Port=2
  wires:
  Sum1/1 -> Product2/2
  Constant4/1 -> Gain/1
  Product/1 -> Product1/1
  Constant3/1 -> Sum/2
  Constant5/1 -> Sum/1
  Constant9/1 -> Cross Product/1
  Gain1/1 -> Product/1
  Dot Product1/1 -> Product5/2
  Product3/1 -> Sum1/1
  Cross Product/1 -> M_P4/1
  Constant1/1 -> Product/2
  Sum2/1 -> Product4/1
  Constant7/1 -> Gain2/1
  Constant/1 -> Gain1/1
  Gain2/1 -> Product5/1
  Gain/1 -> Sum2/2
  Constant2/1 -> Dot Product/2
  Product1/1 -> Product2/1
  Sum/1 -> Product3/1
  Constant6/1 -> Product4/2
  Constant8/1 -> Dot Product1/2
  Product4/1 -> Sum1/2
  Product5/1 -> Sum2/1
  Product2/1 -> Scope/1, Cross Product/2, F_P4/1  "F_P4"
  S_B/1 -> Product3/2, Dot Product1/1, Dot Product/1
  Constant10/1 -> Relational Operator/2
  Relational Operator/1 -> Product6/2
  Product6/1 -> Product1/2
  Dot Product/1 -> Product6/1, Relational Operator/1

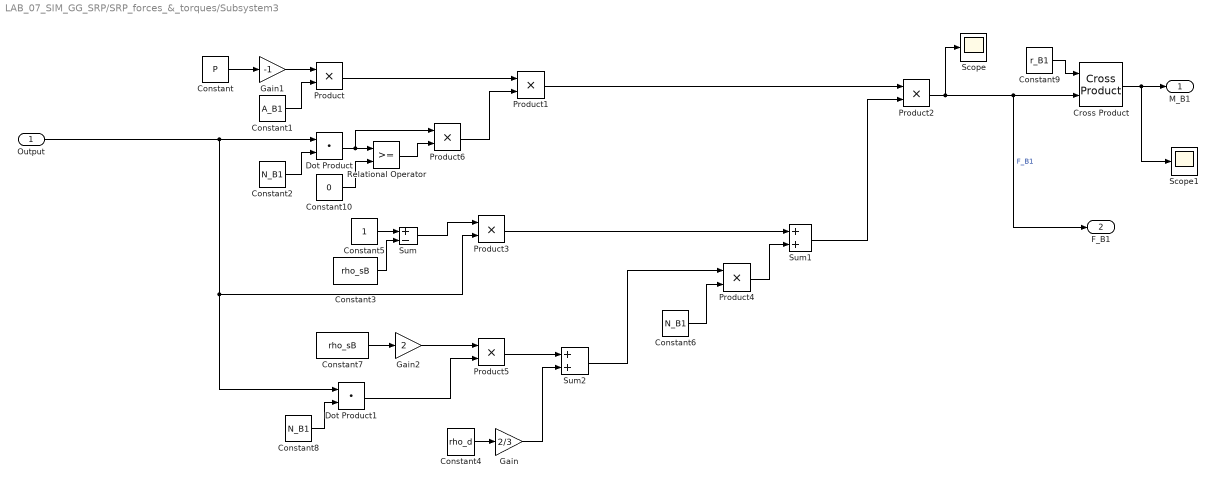
== system LAB_07_SIM_GG_SRP/SRP_forces_&_torques/Subsystem3 ==
  Output : Inport
  Constant : Constant  Value=P
  Constant1 : Constant  Value=A_B1
  Constant10 : Constant  Value=0
  Constant2 : Constant  Value=N_B1
  Constant3 : Constant  Value=rho_sB
  Constant4 : Constant  Value=rho_d
  Constant5 : Constant
  Constant6 : Constant  Value=N_B1
  Constant7 : Constant  Value=rho_sB
  Constant8 : Constant  Value=N_B1
  Constant9 : Constant  Value=r_B1
  Cross Product : matrix_library/Cross Product
  Dot Product : DotProduct  OutDataTypeStr=Inherit: Inherit via internal rule
  Dot Product1 : DotProduct  OutDataTypeStr=Inherit: Inherit via internal rule
  Gain : Gain  Gain=2/3
  Gain1 : Gain  Gain=-1
  Gain2 : Gain  Gain=2
  Product{,1..6} (7 alike) : Product
  Relational Operator : RelationalOperator  OutDataTypeStr=boolean  RndMeth=Simplest  InputSameDT=off
  Scope : Scope
  Scope1 : Scope
  Sum : Sum  Inputs=+-
  Sum1 : Sum
  Sum2 : Sum
  M_B1 : Outport
  F_B1 : Outport  Port=2
  wires:
  Output/1 -> Dot Product/1, Dot Product1/1, Product3/2
  Product2/1 -> F_B1/1, Cross Product/2, Scope/1  "F_B1"
  Product5/1 -> Sum2/1
  Product4/1 -> Sum1/2
  Constant8/1 -> Dot Product1/2
  Constant6/1 -> Product4/2
  Sum/1 -> Product3/1
  Product1/1 -> Product2/1
  Constant2/1 -> Dot Product/2
  Gain/1 -> Sum2/2
  Gain2/1 -> Product5/1
  Constant/1 -> Gain1/1
  Constant7/1 -> Gain2/1
  Sum2/1 -> Product4/1
  Constant1/1 -> Product/2
  Cross Product/1 -> Scope1/1, M_B1/1
  Product3/1 -> Sum1/1
  Gain1/1 -> Product/1
  Constant9/1 -> Cross Product/1
  Constant5/1 -> Sum/1
  Constant3/1 -> Sum/2
  Product/1 -> Product1/1
  Constant4/1 -> Gain/1
  Sum1/1 -> Product2/2
  Constant10/1 -> Relational Operator/2
  Dot Product/1 -> Product6/1, Relational Operator/1
  Dot Product1/1 -> Product5/2
  Relational Operator/1 -> Product6/2
  Product6/1 -> Product1/2

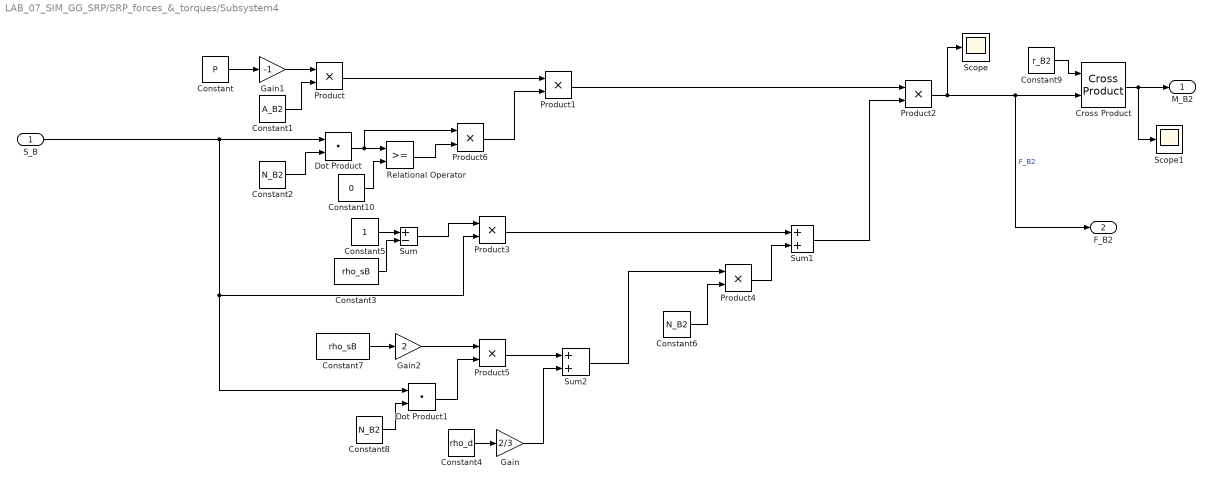
== system LAB_07_SIM_GG_SRP/SRP_forces_&_torques/Subsystem4 ==
  S_B : Inport
  Constant : Constant  Value=P
  Constant1 : Constant  Value=A_B2
  Constant10 : Constant  Value=0
  Constant2 : Constant  Value=N_B2
  Constant3 : Constant  Value=rho_sB
  Constant4 : Constant  Value=rho_d
  Constant5 : Constant
  Constant6 : Constant  Value=N_B2
  Constant7 : Constant  Value=rho_sB
  Constant8 : Constant  Value=N_B2
  Constant9 : Constant  Value=r_B2
  Cross Product : matrix_library/Cross Product
  Dot Product : DotProduct  OutDataTypeStr=Inherit: Inherit via internal rule
  Dot Product1 : DotProduct  OutDataTypeStr=Inherit: Inherit via internal rule
  Gain : Gain  Gain=2/3
  Gain1 : Gain  Gain=-1
  Gain2 : Gain  Gain=2
  Product{,1..6} (7 alike) : Product
  Relational Operator : RelationalOperator  OutDataTypeStr=boolean  RndMeth=Simplest  InputSameDT=off
  Scope : Scope
  Scope1 : Scope
  Sum : Sum  Inputs=+-
  Sum1 : Sum
  Sum2 : Sum
  M_B2 : Outport
  F_B2 : Outport  Port=2
  wires:
  Sum1/1 -> Product2/2
  Constant4/1 -> Gain/1
  Product/1 -> Product1/1
  Constant3/1 -> Sum/2
  Constant5/1 -> Sum/1
  Constant9/1 -> Cross Product/1
  Gain1/1 -> Product/1
  Dot Product1/1 -> Product5/2
  Product3/1 -> Sum1/1
  Cross Product/1 -> Scope1/1, M_B2/1
  Constant1/1 -> Product/2
  Sum2/1 -> Product4/1
  Constant7/1 -> Gain2/1
  Constant/1 -> Gain1/1
  Gain2/1 -> Product5/1
  Gain/1 -> Sum2/2
  Constant2/1 -> Dot Product/2
  Product1/1 -> Product2/1
  Sum/1 -> Product3/1
  Constant6/1 -> Product4/2
  Constant8/1 -> Dot Product1/2
  Product4/1 -> Sum1/2
  Product5/1 -> Sum2/1
  Product2/1 -> Scope/1, Cross Product/2, F_B2/1  "F_B2"
  S_B/1 -> Product3/2, Dot Product1/1, Dot Product/1
  Dot Product/1 -> Product6/1, Relational Operator/1
  Constant10/1 -> Relational Operator/2
  Relational Operator/1 -> Product6/2
  Product6/1 -> Product1/2

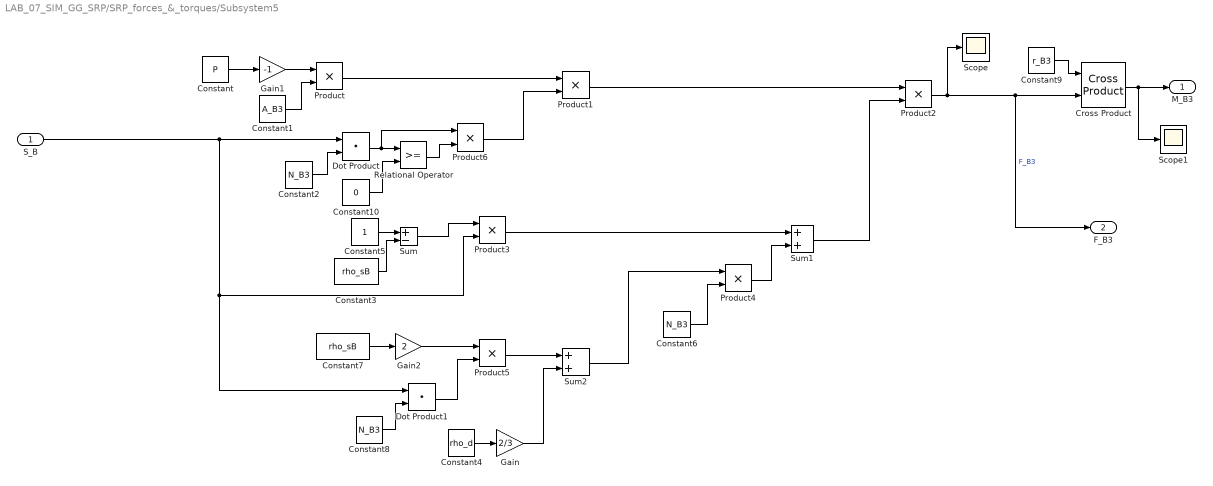
== system LAB_07_SIM_GG_SRP/SRP_forces_&_torques/Subsystem5 ==
  S_B : Inport
  Constant : Constant  Value=P
  Constant1 : Constant  Value=A_B3
  Constant10 : Constant  Value=0
  Constant2 : Constant  Value=N_B3
  Constant3 : Constant  Value=rho_sB
  Constant4 : Constant  Value=rho_d
  Constant5 : Constant
  Constant6 : Constant  Value=N_B3
  Constant7 : Constant  Value=rho_sB
  Constant8 : Constant  Value=N_B3
  Constant9 : Constant  Value=r_B3
  Cross Product : matrix_library/Cross Product
  Dot Product : DotProduct  OutDataTypeStr=Inherit: Inherit via internal rule
  Dot Product1 : DotProduct  OutDataTypeStr=Inherit: Inherit via internal rule
  Gain : Gain  Gain=2/3
  Gain1 : Gain  Gain=-1
  Gain2 : Gain  Gain=2
  Product{,1..6} (7 alike) : Product
  Relational Operator : RelationalOperator  OutDataTypeStr=boolean  RndMeth=Simplest  InputSameDT=off
  Scope : Scope
  Scope1 : Scope
  Sum : Sum  Inputs=+-
  Sum1 : Sum
  Sum2 : Sum
  M_B3 : Outport
  F_B3 : Outport  Port=2
  wires:
  S_B/1 -> Dot Product/1, Dot Product1/1, Product3/2
  Product2/1 -> F_B3/1, Cross Product/2, Scope/1  "F_B3"
  Product5/1 -> Sum2/1
  Product4/1 -> Sum1/2
  Constant8/1 -> Dot Product1/2
  Constant6/1 -> Product4/2
  Sum/1 -> Product3/1
  Product1/1 -> Product2/1
  Constant2/1 -> Dot Product/2
  Gain/1 -> Sum2/2
  Gain2/1 -> Product5/1
  Constant/1 -> Gain1/1
  Constant7/1 -> Gain2/1
  Sum2/1 -> Product4/1
  Constant1/1 -> Product/2
  Cross Product/1 -> Scope1/1, M_B3/1
  Product3/1 -> Sum1/1
  Dot Product1/1 -> Product5/2
  Gain1/1 -> Product/1
  Constant9/1 -> Cross Product/1
  Constant5/1 -> Sum/1
  Constant3/1 -> Sum/2
  Product/1 -> Product1/1
  Constant4/1 -> Gain/1
  Sum1/1 -> Product2/2
  Constant10/1 -> Relational Operator/2
  Relational Operator/1 -> Product6/2
  Product6/1 -> Product1/2
  Dot Product/1 -> Product6/1, Relational Operator/1

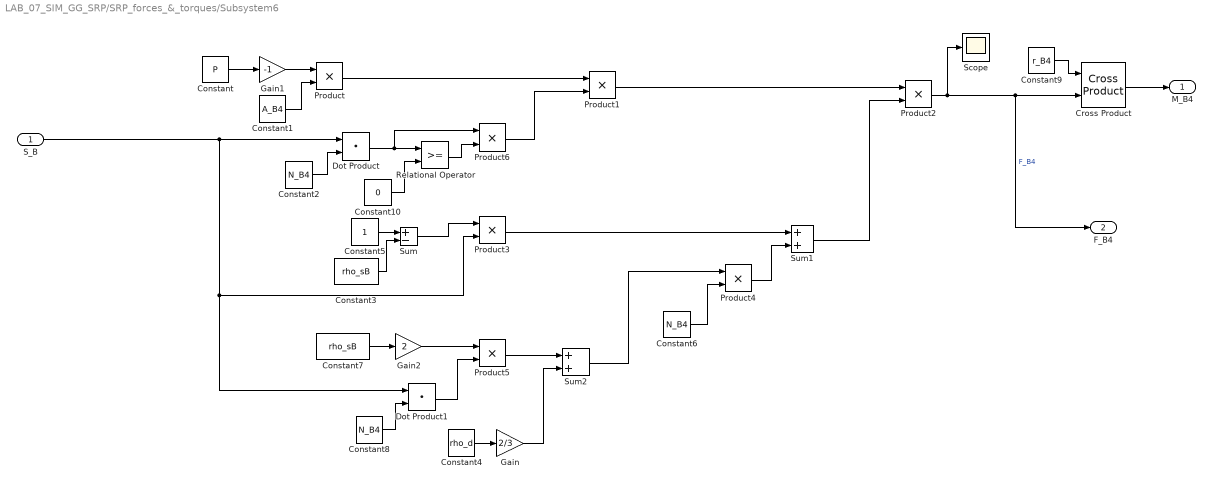
== system LAB_07_SIM_GG_SRP/SRP_forces_&_torques/Subsystem6 ==
  S_B : Inport
  Constant : Constant  Value=P
  Constant1 : Constant  Value=A_B4
  Constant10 : Constant  Value=0
  Constant2 : Constant  Value=N_B4
  Constant3 : Constant  Value=rho_sB
  Constant4 : Constant  Value=rho_d
  Constant5 : Constant
  Constant6 : Constant  Value=N_B4
  Constant7 : Constant  Value=rho_sB
  Constant8 : Constant  Value=N_B4
  Constant9 : Constant  Value=r_B4
  Cross Product : matrix_library/Cross Product
  Dot Product : DotProduct  OutDataTypeStr=Inherit: Inherit via internal rule
  Dot Product1 : DotProduct  OutDataTypeStr=Inherit: Inherit via internal rule
  Gain : Gain  Gain=2/3
  Gain1 : Gain  Gain=-1
  Gain2 : Gain  Gain=2
  Product{,1..6} (7 alike) : Product
  Relational Operator : RelationalOperator  OutDataTypeStr=boolean  RndMeth=Simplest  InputSameDT=off
  Scope : Scope
  Sum : Sum  Inputs=+-
  Sum1 : Sum
  Sum2 : Sum
  M_B4 : Outport
  F_B4 : Outport  Port=2
  wires:
  Sum1/1 -> Product2/2
  Constant4/1 -> Gain/1
  Product/1 -> Product1/1
  Constant3/1 -> Sum/2
  Constant5/1 -> Sum/1
  Constant9/1 -> Cross Product/1
  Gain1/1 -> Product/1
  Dot Product1/1 -> Product5/2
  Product3/1 -> Sum1/1
  Cross Product/1 -> M_B4/1
  Constant1/1 -> Product/2
  Sum2/1 -> Product4/1
  Constant7/1 -> Gain2/1
  Constant/1 -> Gain1/1
  Gain2/1 -> Product5/1
  Gain/1 -> Sum2/2
  Constant2/1 -> Dot Product/2
  Product1/1 -> Product2/1
  Sum/1 -> Product3/1
  Constant6/1 -> Product4/2
  Constant8/1 -> Dot Product1/2
  Product4/1 -> Sum1/2
  Product5/1 -> Sum2/1
  Product2/1 -> Scope/1, Cross Product/2, F_B4/1  "F_B4"
  S_B/1 -> Product3/2, Dot Product1/1, Dot Product/1
  Constant10/1 -> Relational Operator/2
  Relational Operator/1 -> Product6/2
  Product6/1 -> Product1/2
  Dot Product/1 -> Product6/1, Relational Operator/1

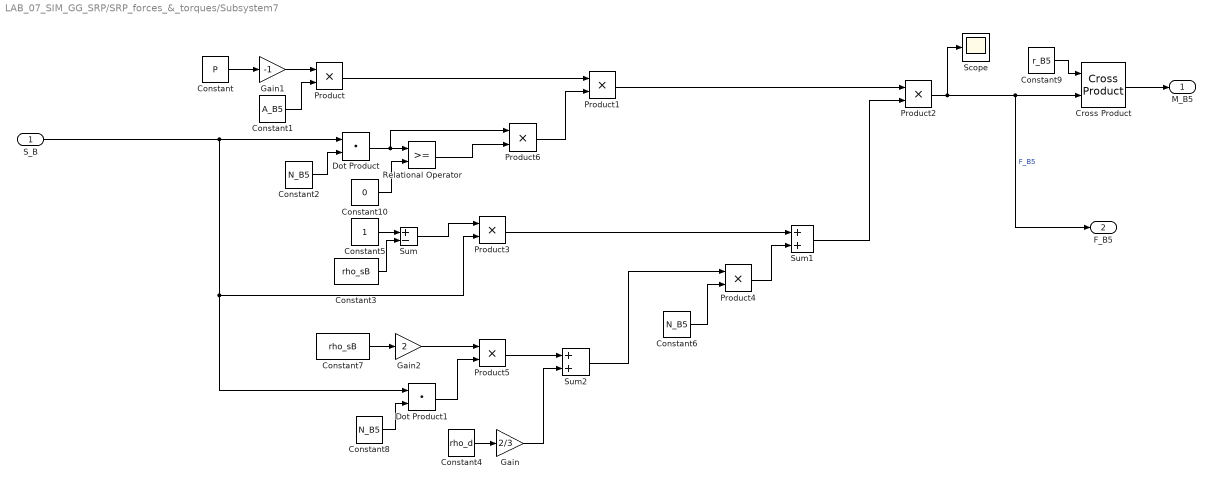
== system LAB_07_SIM_GG_SRP/SRP_forces_&_torques/Subsystem7 ==
  S_B : Inport
  Constant : Constant  Value=P
  Constant1 : Constant  Value=A_B5
  Constant10 : Constant  Value=0
  Constant2 : Constant  Value=N_B5
  Constant3 : Constant  Value=rho_sB
  Constant4 : Constant  Value=rho_d
  Constant5 : Constant
  Constant6 : Constant  Value=N_B5
  Constant7 : Constant  Value=rho_sB
  Constant8 : Constant  Value=N_B5
  Constant9 : Constant  Value=r_B5
  Cross Product : matrix_library/Cross Product
  Dot Product : DotProduct  OutDataTypeStr=Inherit: Inherit via internal rule
  Dot Product1 : DotProduct  OutDataTypeStr=Inherit: Inherit via internal rule
  Gain : Gain  Gain=2/3
  Gain1 : Gain  Gain=-1
  Gain2 : Gain  Gain=2
  Product{,1..6} (7 alike) : Product
  Relational Operator : RelationalOperator  OutDataTypeStr=boolean  RndMeth=Simplest  InputSameDT=off
  Scope : Scope
  Sum : Sum  Inputs=+-
  Sum1 : Sum
  Sum2 : Sum
  M_B5 : Outport
  F_B5 : Outport  Port=2
  wires:
  S_B/1 -> Dot Product/1, Dot Product1/1, Product3/2
  Product2/1 -> F_B5/1, Cross Product/2, Scope/1  "F_B5"
  Product5/1 -> Sum2/1
  Product4/1 -> Sum1/2
  Constant8/1 -> Dot Product1/2
  Constant6/1 -> Product4/2
  Sum/1 -> Product3/1
  Product1/1 -> Product2/1
  Constant2/1 -> Dot Product/2
  Gain/1 -> Sum2/2
  Gain2/1 -> Product5/1
  Constant/1 -> Gain1/1
  Constant7/1 -> Gain2/1
  Sum2/1 -> Product4/1
  Constant1/1 -> Product/2
  Cross Product/1 -> M_B5/1
  Product3/1 -> Sum1/1
  Dot Product1/1 -> Product5/2
  Gain1/1 -> Product/1
  Constant9/1 -> Cross Product/1
  Constant5/1 -> Sum/1
  Constant3/1 -> Sum/2
  Product/1 -> Product1/1
  Constant4/1 -> Gain/1
  Sum1/1 -> Product2/2
  Constant10/1 -> Relational Operator/2
  Relational Operator/1 -> Product6/2
  Product6/1 -> Product1/2
  Dot Product/1 -> Product6/1, Relational Operator/1

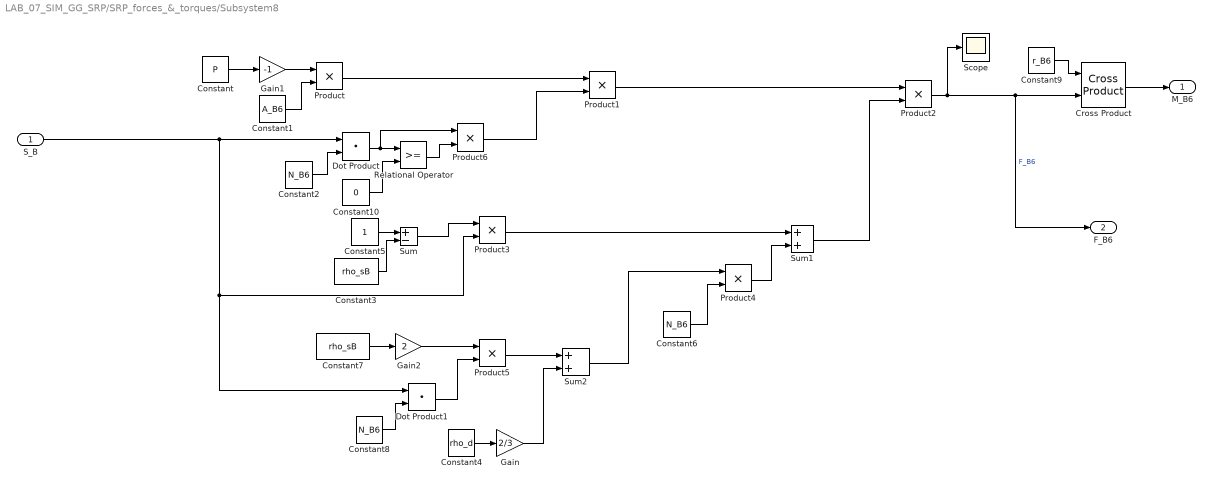
== system LAB_07_SIM_GG_SRP/SRP_forces_&_torques/Subsystem8 ==
  S_B : Inport
  Constant : Constant  Value=P
  Constant1 : Constant  Value=A_B6
  Constant10 : Constant  Value=0
  Constant2 : Constant  Value=N_B6
  Constant3 : Constant  Value=rho_sB
  Constant4 : Constant  Value=rho_d
  Constant5 : Constant
  Constant6 : Constant  Value=N_B6
  Constant7 : Constant  Value=rho_sB
  Constant8 : Constant  Value=N_B6
  Constant9 : Constant  Value=r_B6
  Cross Product : matrix_library/Cross Product
  Dot Product : DotProduct  OutDataTypeStr=Inherit: Inherit via internal rule
  Dot Product1 : DotProduct  OutDataTypeStr=Inherit: Inherit via internal rule
  Gain : Gain  Gain=2/3
  Gain1 : Gain  Gain=-1
  Gain2 : Gain  Gain=2
  Product{,1..6} (7 alike) : Product
  Relational Operator : RelationalOperator  OutDataTypeStr=boolean  RndMeth=Simplest  InputSameDT=off
  Scope : Scope
  Sum : Sum  Inputs=+-
  Sum1 : Sum
  Sum2 : Sum
  M_B6 : Outport
  F_B6 : Outport  Port=2
  wires:
  Sum1/1 -> Product2/2
  Constant4/1 -> Gain/1
  Product/1 -> Product1/1
  Constant3/1 -> Sum/2
  Constant5/1 -> Sum/1
  Constant9/1 -> Cross Product/1
  Gain1/1 -> Product/1
  Dot Product1/1 -> Product5/2
  Product3/1 -> Sum1/1
  Cross Product/1 -> M_B6/1
  Constant1/1 -> Product/2
  Sum2/1 -> Product4/1
  Constant7/1 -> Gain2/1
  Constant/1 -> Gain1/1
  Gain2/1 -> Product5/1
  Gain/1 -> Sum2/2
  Constant2/1 -> Dot Product/2
  Product1/1 -> Product2/1
  Sum/1 -> Product3/1
  Constant6/1 -> Product4/2
  Constant8/1 -> Dot Product1/2
  Product4/1 -> Sum1/2
  Product5/1 -> Sum2/1
  Product2/1 -> Scope/1, Cross Product/2, F_B6/1  "F_B6"
  S_B/1 -> Product3/2, Dot Product1/1, Dot Product/1
  Constant10/1 -> Relational Operator/2
  Relational Operator/1 -> Product6/2
  Product6/1 -> Product1/2
  Dot Product/1 -> Product6/1, Relational Operator/1

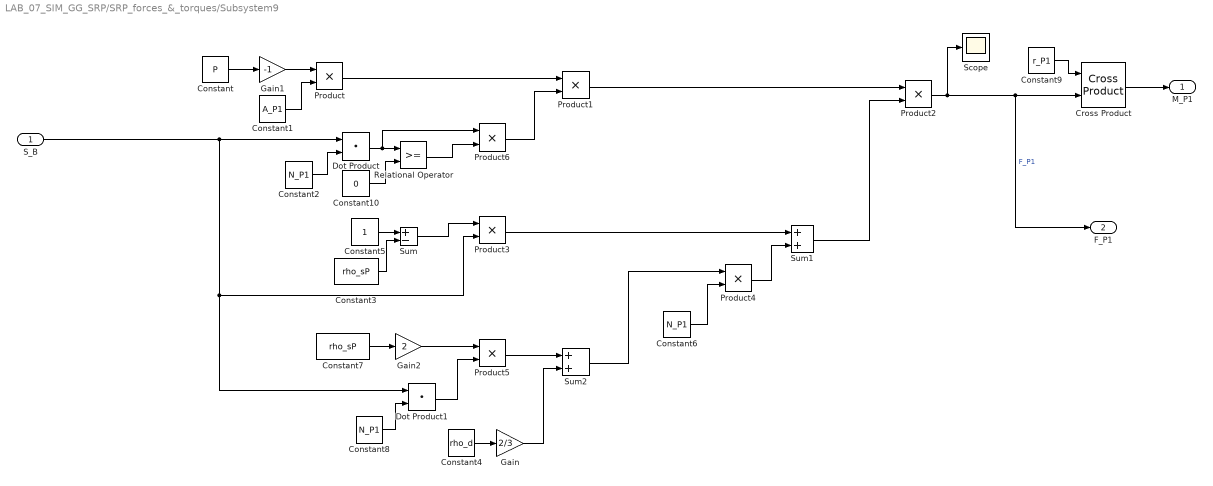
== system LAB_07_SIM_GG_SRP/SRP_forces_&_torques/Subsystem9 ==
  S_B : Inport
  Constant : Constant  Value=P
  Constant1 : Constant  Value=A_P1
  Constant10 : Constant  Value=0
  Constant2 : Constant  Value=N_P1
  Constant3 : Constant  Value=rho_sP
  Constant4 : Constant  Value=rho_d
  Constant5 : Constant
  Constant6 : Constant  Value=N_P1
  Constant7 : Constant  Value=rho_sP
  Constant8 : Constant  Value=N_P1
  Constant9 : Constant  Value=r_P1
  Cross Product : matrix_library/Cross Product
  Dot Product : DotProduct  OutDataTypeStr=Inherit: Inherit via internal rule
  Dot Product1 : DotProduct  OutDataTypeStr=Inherit: Inherit via internal rule
  Gain : Gain  Gain=2/3
  Gain1 : Gain  Gain=-1
  Gain2 : Gain  Gain=2
  Product{,1..6} (7 alike) : Product
  Relational Operator : RelationalOperator  OutDataTypeStr=boolean  RndMeth=Simplest  InputSameDT=off
  Scope : Scope
  Sum : Sum  Inputs=+-
  Sum1 : Sum
  Sum2 : Sum
  M_P1 : Outport
  F_P1 : Outport  Port=2
  wires:
  S_B/1 -> Dot Product/1, Dot Product1/1, Product3/2
  Product2/1 -> F_P1/1, Cross Product/2, Scope/1  "F_P1"
  Product5/1 -> Sum2/1
  Product4/1 -> Sum1/2
  Constant8/1 -> Dot Product1/2
  Constant6/1 -> Product4/2
  Sum/1 -> Product3/1
  Product1/1 -> Product2/1
  Constant2/1 -> Dot Product/2
  Gain/1 -> Sum2/2
  Gain2/1 -> Product5/1
  Constant/1 -> Gain1/1
  Constant7/1 -> Gain2/1
  Sum2/1 -> Product4/1
  Constant1/1 -> Product/2
  Cross Product/1 -> M_P1/1
  Product3/1 -> Sum1/1
  Dot Product1/1 -> Product5/2
  Gain1/1 -> Product/1
  Constant9/1 -> Cross Product/1
  Constant5/1 -> Sum/1
  Constant3/1 -> Sum/2
  Product/1 -> Product1/1
  Constant4/1 -> Gain/1
  Sum1/1 -> Product2/2
  Constant10/1 -> Relational Operator/2
  Relational Operator/1 -> Product6/2
  Product6/1 -> Product1/2
  Dot Product/1 -> Product6/1, Relational Operator/1

== system LAB_07_SIM_GG_SRP/Subsystem/Check_Orthogonality_S ==
  S : Inport
  MATLAB Function1 : MATLAB Function  TreatAsAtomicUnit=on
  Scope3 : Scope
  wires:
  MATLAB Function1/1(perp_flag) -> Scope3/1
  S/1 -> MATLAB Function1/1(S)

== system LAB_07_SIM_GG_SRP/Subsystem/Check_Orthogonality_V ==
  V : Inport
  MATLAB Function2 : MATLAB Function  TreatAsAtomicUnit=on
  Scope4 : Scope
  wires:
  MATLAB Function2/1(perpp_flag) -> Scope4/1
  V/1 -> MATLAB Function2/1(S)

== system LAB_07_SIM_GG_SRP/Subsystem/DCM ==
  note: A
  omega : Inport
  Determinant Chech fo Validation : Subsystem
  Gain1 : Gain  Gain=-1
  Integrator1 : Integrator  InitialCondition=A0
  Product2 : Product  Multiplication=Matrix(*)
  Scope1 : Scope
  Scope2 : Scope
  Subsystem : Subsystem
  matrix of omega cross prod : Subsystem
  DCM : Outport
  wires:
  Integrator1/1 -> Subsystem/1(A1), Scope2/1, Determinant Chech fo Validation/1(DCM), DCM/1
  matrix of omega cross prod/1(Out1) -> Product2/1
  Product2/1 -> Gain1/1  "A_dot"
  omega/1 -> matrix of omega cross prod/1(om)
  Gain1/1 -> Integrator1/1, Scope1/1
  Subsystem/1(A_orthonormalized1) -> Product2/2

== system LAB_07_SIM_GG_SRP/Subsystem/norm ==
  Input : Inport
  Demux : Demux  Outputs=3
  Sqrt : Sqrt
  Square : Math  Operator=square
  Square1 : Math  Operator=square
  Square2 : Math  Operator=square
  Sum : Sum  Inputs=+++
  Output : Outport
  wires:
  Square/1 -> Sum/1
  Square1/1 -> Sum/2
  Square2/1 -> Sum/3
  Sum/1 -> Sqrt/1
  Input/1 -> Demux/1
  Sqrt/1 -> Output/1
  Demux/1 -> Square/1
  Demux/2 -> Square1/1
  Demux/3 -> Square2/1

== system LAB_07_SIM_GG_SRP/Subsystem/norm1 ==
  Input : Inport
  Demux : Demux  Outputs=3
  Sqrt : Sqrt
  Square : Math  Operator=square
  Square1 : Math  Operator=square
  Square2 : Math  Operator=square
  Sum : Sum  Inputs=+++
  Output : Outport
  wires:
  Square/1 -> Sum/1
  Square1/1 -> Sum/2
  Square2/1 -> Sum/3
  Sum/1 -> Sqrt/1
  Input/1 -> Demux/1
  Sqrt/1 -> Output/1
  Demux/1 -> Square/1
  Demux/2 -> Square1/1
  Demux/3 -> Square2/1
